simulink model "uGrid_1PH_hd_ATD2"  (R2018a)
settings: Solver=VariableStepAuto  StartTime=0.0  StopTime=.5  FixedStep=1e-6  MaxStep=1e-4  RelTol=1e-3
PreLoadFcn:
  | SimulinkInit
InitFcn:
  | SimulinkInit
StopFcn:
  | EndingScript
values from neighbouring files (symbols this model uses):
  ssAl = [-2.49999998232 0 0 0 376.789751319 0 -3.33333337039 0 0 376.789751319 0 0 ... (25 elements, 5x5)]    [modeloElectrico.mat]
  ssBl = [24.9999999997 0 0 0 0 0 33.333333333 0 0 0 0 0 ... (15 elements, 5x3)]    [modeloElectrico.mat]
  ssCl = [-0.229841748304 -0.00828937452901 0.991710625471 0 -0.229841748304 0.991710625471 -0.00828937452901 0 0.770158251696 -0.00828937452901 -0.00828937452901 0 ... (20 elements, 4x5)]    [modeloElectrico.mat]
  Tao1 = 0.5    [SimulinkInit.m]    (also in modeloDiesel_dotros.mat)
undefined symbols (not defined in the file or in its folder): G, GF, Ion, Lithium, ss1, ss2
libraries: powerlib x59, dsparch4 x12, truetime x12, powerlib_meascontrol x4, simulink x2, electricdrivelib x1
(part 1 of 2)
settings Model: Creator=erich  LastModifiedBy=cmparedes
settings CodeAppCC: StateflowObjectComments=on
settings SimscapeCC: SimscapeNormalizeSystem=off

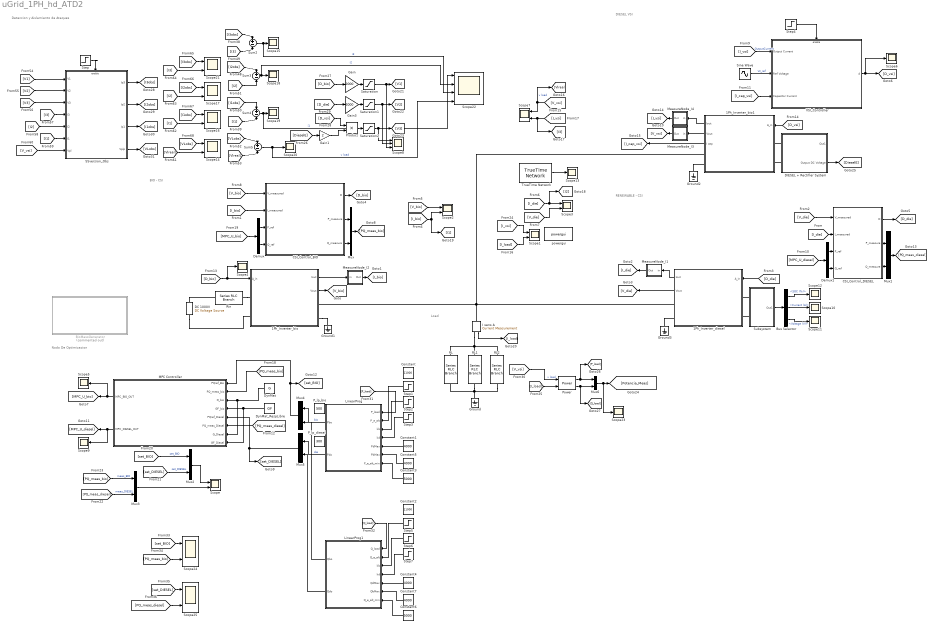
== system uGrid_1PH_hd_ATD2 ==
  note: Deteccion y Aislamiento de Ataques
  note: DIESEL VSI
  note: Load
  note: BIO - CSI
  note: RENEWABLE - CSI
  note: Nodo De Optimizacion
  1Ph_Inverter_bio : Subsystem  mask{st_time=0, f_sw=12000, samp_f=1e-6}
      mask prompts: st_time "Tiempo muerto (Start)"; f_sw "Switching frequency"; samp_f "samplig"
      mask Display:
      | port_label('input', 1, 'd', 'texmode', 'on')
      | 
      | port_label('lconn', 1, 'DC +')
      | port_label('lconn', 2, 'DC -')
      | 
      | 
      | port_label('rconn', 1, 'V_{out+}')
      | port_label('rconn', 2, 'B_{out-}')
      | 
      | 
      | port_label('output', 1, 'I_{out}', 'texmode', 'on')
      | port_label('output', 2, 'V_{out}', 'texmode', 'on')
      | 
      | plot([0.1 .9], [0.1 .9])
      | plot([0.2 .4], [.7 .7])
      | plot([0.2 .24], [.65 .65])
      | plot([0.28 .32], [.65 .65])
      | plot([0.36 .40], [.65 .65])
      | 
      | plot([.5:.01:.7], .25+sin(30*[.2:.01:.4])/10)
  1Ph_Inverter_bio1 : Subsystem  mask{st_time=0, f_sw=12000, samp_f=1e-6}
      mask prompts: st_time "Tiempo muerto (Start)"; f_sw "Switching frequency"; samp_f "samplig"
      mask Display:
      | port_label('input', 1, 'd', 'texmode', 'on')
      | 
      | port_label('lconn', 1, 'DC +')
      | port_label('lconn', 2, 'DC -')
      | 
      | 
      | port_label('rconn', 1, 'V_{out+}')
      | port_label('rconn', 2, 'B_{out-}')
      | 
      | 
      | port_label('output', 1, 'I_{out}', 'texmode', 'on')
      | port_label('output', 2, 'V_{out}', 'texmode', 'on')
      | port_label('output', 3, 'I_{cap}', 'texmode', 'on')
      | 
      | plot([0.1 .9], [0.1 .9])
      | plot([0.2 .4], [.7 .7])
      | plot([0.2 .24], [.65 .65])
      | plot([0.28 .32], [.65 .65])
      | plot([0.36 .40], [.65 .65])
      | 
      | plot([.5:.01:.7], .25+sin(30*[.2:.01:.4])/10)
  1Ph_Inverter_diesel : Subsystem  mask{st_time=0, f_sw=12000, samp_f=1e-6}
      mask prompts: st_time "Tiempo muerto (Start)"; f_sw "Switching frequency"; samp_f "Sampling frequency"
      mask Display:
      | port_label('input', 1, 'd', 'texmode', 'on')
      | 
      | port_label('lconn', 1, 'DC +')
      | port_label('lconn', 2, 'DC -')
      | 
      | 
      | port_label('rconn', 1, 'V_{out+}')
      | port_label('rconn', 2, 'B_{out-}')
      | 
      | 
      | port_label('output', 1, 'I_{out}', 'texmode', 'on')
      | port_label('output', 2, 'V_{out}', 'texmode', 'on')
      | 
      | plot([0.1 .9], [0.1 .9])
      | plot([0.2 .4], [.7 .7])
      | plot([0.2 .24], [.65 .65])
      | plot([0.28 .32], [.65 .65])
      | plot([0.36 .40], [.65 .65])
      | 
      | plot([.5:.01:.7], .25+sin(30*[.2:.01:.4])/10)
  BioMassGenerator : Subsystem  Commented=on
  Bus Selector : BusSelector  OutputSignals=SOC (%),Current (A),Voltage (V)
  CSI_Control_BIO : Subsystem
  CSI_Control_DIESEL : Subsystem
  Constant : Constant  Value=11000
  Constant{1,4..5,7} (4 alike) : Constant  Value=4000
  Constant2 : Constant  Value=11000
  Constant3 : Constant  Value=5000
  Constant6 : Constant  Value=5000
  DC 1000V : powerlib/Electrical Sources/DC Voltage Source  Amplitude=1000  Measurements=None
  DIESEL + Rectifier System : Subsystem
  Demux : Demux  Outputs=2
  Demux1 : Demux  Outputs=2
  DynMat : Constant  Value=G
  DynMat_RespLibre : Constant  Value=GF
  Gain : Gain  Gain=2000
  Gain1 : Gain  Gain=2
  Gain3 : Gain  Gain=2000
  Ground{,1..3} (4 alike) : powerlib/Elements/Ground  LConnTagsString=a
  I sens A : powerlib/Measurements/Current Measurement  PhasorSimulation=off  OutputType=Complex  PSBequivalent=0
  LinearProg : MATLAB Function  TreatAsAtomicUnit=on  SystemSampleTime=1e-3
  LinearProg1 : MATLAB Function  TreatAsAtomicUnit=on  SystemSampleTime=1e-3
  MPC Controller : Subsystem
  MeasureNode_I1 : Subsystem
  MeasureNode_I2 : Subsystem
  MeasureNode_I3 : Subsystem
  MeasureNode_I4 : Subsystem
  Mux{,1..6} (7 alike) : Mux  Inputs=2
  P_lp_bio : Constant  Value=500
  P_lp_diesel : Constant  Value=300
  Power : powerlib_meascontrol/Measurements/Power  Freq=60  Vinit=[1, 0]  Iinit=[1, 0]  Ts=0
      settings: SourceProductName=Simscape Power Systems
  Product : Product
  RL : powerlib/Elements/Series RLC Branch  LConnTagsString=__new0  RConnTagsString=__new0  BranchType=R  Resistance=10  Inductance=500e-3  SetiL0=off  InitialCurrent=0  Capacitance=100e-6  Setx0=off  InitialVoltage=0  Measurements=None
  RL1 : powerlib/Elements/Series RLC Branch  LConnTagsString=__new0  RConnTagsString=__new0  BranchType=RL  Resistance=10  Inductance=5.2  SetiL0=off  InitialCurrent=0  Capacitance=100e-6  Setx0=off  InitialVoltage=0  Measurements=None
  RL2 : powerlib/Elements/Series RLC Branch  LConnTagsString=__new0  RConnTagsString=__new0  BranchType=C  Resistance=30  Inductance=500e-3  SetiL0=off  InitialCurrent=0  Capacitance=2000e-6  Setx0=off  InitialVoltage=0  Measurements=None
  Rin : powerlib/Elements/Series RLC Branch  LConnTagsString=__new0  RConnTagsString=__new0  BranchType=R  Resistance=.001  Inductance=0  SetiL0=off  InitialCurrent=0  Capacitance=0  Setx0=off  InitialVoltage=0  Measurements=None
  SSversion_Obs : Subsystem
  Saturation : Saturate  UpperLimit=1000  LowerLimit=-1000
  Saturation1 : Saturate  UpperLimit=1000  LowerLimit=-1000
  Saturation2 : Saturate  UpperLimit=1000  LowerLimit=-1000
  Scope{,1..3,7,14,16..17,21,24..25} (11 alike) : Scope  NumInputPorts=2
  Scope{4..6,9..13,15,18..20,23} (13 alike) : Scope
  Scope22 : Scope  NumInputPorts=4
  Scope8 : Scope  NumInputPorts=3
  Sine Wave : Sin  Amplitude=170  Frequency=2*pi*60  SampleTime=0
  Step : Step  Time=0  SampleTime=0
  Step1 : Step  Time=0.3  Before=20000  After=5000  SampleTime=0
  Step2 : Step  Time=.6  Before=1.2  After=.4  SampleTime=0
  Step3 : Step  Before=.7  After=.7  SampleTime=0
  Step4 : Step  Time=10e-3  SampleTime=0
  Step5 : Step  Time=.3  Before=20000  After=5000  SampleTime=0
  Step6 : Step  Time=.6  Before=1.2  After=.4  SampleTime=0
  Step7 : Step  Before=.7  After=.7  SampleTime=0
  Subsystem : Subsystem
  Sum{2..5} (4 alike) : Sum  Inputs=+-
  TrueTime Network : truetime/TrueTime Network  nwtype=CSMA/CD (Ethernet)  nwnbr=1  nnodes=10  rate=8*1e9  minsize=512  lossprob=0  seed=0  bandwidths=[0.5 0.5]  slotsize=512  schedule=[1 1 2]  memsize=80000  buftype=Common buffer  overflow=Retransmit  dynSchedule=0  miniSlotSize=0  NIT=0  QSortMode=FIFO  sync=0  irtSchedule=0  nrtLength=0  nodeGraph=0  scheduleoutput=on
  VSI_Controller : Subsystem
  powergui : powerlib/powergui  Priority=1  SimulationMode=Continuous  SampleTime=50e-6  frequency=60  Iterations=50  frequencyindice=0  Pbase=100e6  ErrMax=1e-4  UnitsV=kV  UnitsW=MW  buscounter=0  FunctionMessages=off  echomessages=off  EnableUseOfTLC=off  CurrentSourceSwitches=off  DisableSnubberDevices=off  DisableRonSwitches=off  DisableVfSwitches=off  DisplayEquations=off  SolverType=Tustin/Backward Euler (TBE)  Interpol=off  ExternalGateDelay=off  methode=off  Ts=100  x0status=blocks  SPID=on  SwTol=0  HookPort=off  RestoreLinks=warning  ResistiveCurrentMeasurement=off  Frange=[0:2:500]  Ylog=off  Xlog=on  ShowGrid=off  save=off  variable=ZData  structure=0  ZoomFFT=off  StartTime=0.0  cycles=1  DisplayStyle=1  fundamental=60  FreqAxis=off  MaxFrequency=1000  frequencyindicesteady=1  RmsSteady=1  display=off
  wires:
  [D_bio] -> Scope4/1, 1Ph_Inverter_bio/1(A_in)
  [D_die] -> 1Ph_Inverter_diesel/1(A_in)
  [I_bio] -> [I1], Scope2/2
  [V_bio] -> Scope2/1
  [I_die] -> [I2], Scope3/1
  [V_die] -> Scope3/2
  1Ph_Inverter_bio/1(Iout) -> MeasureNode_I2/1(in)
  1Ph_Inverter_bio/2(Vout) -> [V_bio]
  1Ph_Inverter_diesel/1(Iout) -> MeasureNode_I1/1(in)
  1Ph_Inverter_diesel/2(Vout) -> [V_die]
  CSI_Control_BIO/1(D) -> [D_bio]
  [I_bio] -> CSI_Control_BIO/2(I_measured)
  [V_bio] -> CSI_Control_BIO/1(V_measured)
  CSI_Control_DIESEL/1(D) -> [D_die]
  [I_die] -> CSI_Control_DIESEL/2(I_measured)
  [V_die] -> CSI_Control_DIESEL/1(V_measured)
  [I_vsi] -> Scope1/1
  [I_load] -> Scope1/2
  Mux/1 -> [PQ_meas_bio]
  [MPC_U_bio] -> Demux/1
  [MPC_U_diesel] -> Demux1/1
  Mux1/1 -> [PQ_meas_diesel]
  [set_DIESEL] -> Mux2/2  "set_DIESEL"
  [set_BIO] -> Mux2/1  "set_BIO"
  Mux2/1 -> Scope/1
  Mux3/1 -> Scope/2
  [PQ_meas_diesel] -> Mux3/2  "meas_DIESEL"
  [PQ_meas_bio] -> Mux3/1  "meas_BIO"
  CSI_Control_BIO/2(P_measure) -> Mux/1
  CSI_Control_BIO/3(Q_measure) -> Mux/2
  CSI_Control_DIESEL/2(P_measure) -> Mux1/1
  CSI_Control_DIESEL/3(Q_measure) -> Mux1/2
  Demux1/1 -> CSI_Control_DIESEL/3(P_ref)
  Demux1/2 -> CSI_Control_DIESEL/4(Q_ref)
  Demux/1 -> CSI_Control_BIO/3(P_ref)
  Demux/2 -> CSI_Control_BIO/4(Q_ref)
  DynMat_RespLibre/1 -> MPC Controller/4(GF_bio), MPC Controller/8(GF_Diesel)
  DynMat/1 -> MPC Controller/3(G_bio), MPC Controller/7(G_Diesel)
  MPC Controller/2(MPC_DIESEL_OUT) -> [MPC_U_diesel], Scope9/1
  MPC Controller/1(MPC_BIO_OUT) -> Scope5/1, [MPC_U_bio]
  [PQ_meas_bio] -> MPC Controller/2(PQ_meas_bio)
  [PQ_meas_diesel] -> MPC Controller/6(PQ_meas_Diesel)
  Constant3/1 -> LinearProg/7(P_e_alt_min)
  Constant5/1 -> LinearProg/6(PbMax)
  Step2/1 -> LinearProg/3(kb)
  Step3/1 -> LinearProg/4(kd)
  Constant1/1 -> LinearProg/5(PdMax)
  Step1/1 -> LinearProg/2(P_e_alt)
  Mux5/1 -> [set_DIESEL], MPC Controller/5(PQref_Diesel)
  Mux4/1 -> MPC Controller/1(PQref_Bio), [set_BIO]
  VSI_Controller/1(d) -> Scope6/1, [D_vsi]
  [I_vsi] -> VSI_Controller/1(Output Current)  "OutputCurrent"
  Sine Wave/1 -> VSI_Controller/2(Ref Voltage)  "Vc_ref"
  [I_cap_vsi] -> VSI_Controller/3(Capacitor Current)
  1Ph_Inverter_bio1/3(I cap) -> [I_cap_vsi]
  [D_vsi] -> 1Ph_Inverter_bio1/1(A_in)
  1Ph_Inverter_bio1/2(Vout) -> MeasureNode_I3/1(in)
  [V_vsi] -> [Vlreal], Scope7/1  "v load"
  [I_vsi] -> [I3], Scope7/2
  [D_bio] -> Gain/1
  Gain/1 -> Saturation/1
  Saturation/1 -> [V1], Scope8/3
  Saturation1/1 -> Scope8/2, [V2]
  Saturation2/1 -> [V3], Scope8/1
  Product/1 -> Saturation2/1
  Sum2/1 -> Scope22/3, Scope15/1  "i3"
  [I3] -> Sum2/2
  Sum4/1 -> Scope22/1, Scope19/1  "i1"
  [VLobs] -> Sum5/1
  [I2obs] -> Sum3/1
  [I1] -> Sum4/2
  Sum3/1 -> Scope22/2, Scope18/1  "i2"
  [I1obs] -> Sum4/1
  [Vlreal] -> Sum5/2
  Sum5/1 -> Scope22/4, Scope20/1  "v load"
  [I2] -> Sum3/2
  [I3obs] -> Sum2/1
  [D_vsi] -> Product/1
  [V1] -> SSversion_Obs/1(V1)
  [V2] -> SSversion_Obs/2(V2)
  [V3] -> SSversion_Obs/3(V3)
  [I3] -> SSversion_Obs/4(I3)
  [I2] -> SSversion_Obs/5(I2)
  [I1] -> SSversion_Obs/6(I1)
  [V_vsi] -> SSversion_Obs/7(Vpl)
  [I3obs] -> Scope21/1
  [I2obs] -> Scope17/1
  [I2] -> Scope17/2
  [I1] -> Scope16/2
  [Vlreal] -> Scope14/2
  [VLobs] -> Scope14/1
  [I1obs] -> Scope16/1
  [I3] -> Scope21/2
  SSversion_Obs/1(Ip3) -> [I3obs]
  SSversion_Obs/2(Ip2) -> [I2obs]
  SSversion_Obs/3(Ip1) -> [I1obs]
  SSversion_Obs/4(Vplp) -> [VLobs]
  MeasureNode_I2/1(Out) -> [I_bio]
  MeasureNode_I1/1(Out) -> [I_die]
  MeasureNode_I4/1(Out) -> [I_vsi]
  1Ph_Inverter_bio1/1(Iout) -> MeasureNode_I4/1(in)
  I sens A/1 -> [I_load]
  MeasureNode_I3/1(Out) -> [V_vsi]
  [DieselE] -> Gain1/1
  Step/1 -> SSversion_Obs/Enable
  DIESEL + Rectifier System/2(Output DC Voltage) -> [DieselE]
  Bus Selector/2 -> Scope10/1  "<Current (A)>"
  Bus Selector/1 -> Scope12/1  "<SOC (%)>"
  Bus Selector/3 -> Scope11/1  "<Voltage (V)>"
  Subsystem/1(Out1) -> Bus Selector/1
  Step4/1 -> VSI_Controller/Enable
  Gain3/1 -> Saturation1/1
  [D_die] -> Gain3/1
  Gain1/1 -> Product/2
  TrueTime Network/1 -> Scope13/1
  Power/2 -> [Q_load], Mux6/2
  [I_load] -> Power/2
  Mux6/1 -> Scope23/1, [Potencia_Meas]
  [V_vsi] -> Power/1  "v load"
  Power/1 -> [P_load], Mux6/1
  Constant4/1 -> LinearProg1/5(QdMax)
  Step5/1 -> LinearProg1/2(Q_e_alt)
  Constant7/1 -> LinearProg1/6(QbMax)
  Step6/1 -> LinearProg1/3(kb)
  Step7/1 -> LinearProg1/4(kd)
  Constant6/1 -> LinearProg1/7(Q_e_alt_min)
  [P_load] -> LinearProg/1(P_load)
  [Q_load] -> LinearProg1/1(Q_load)
  LinearProg/1(Pbo) -> Mux4/1  "bio"
  LinearProg/2(Pdo) -> Mux5/1  "die"
  LinearProg1/1(Qbo) -> Mux4/2
  LinearProg1/2(Qdo) -> Mux5/2
  [set_BIO] -> Scope24/1
  [PQ_meas_bio] -> Scope24/2
  [set_DIESEL] -> Scope25/1
  [PQ_meas_diesel] -> Scope25/2
  connections:
  RL/LConn1 -- I sens A/RConn1 -- RL2/LConn1 -- RL1/LConn1
  Ground/LConn1 -- RL1/RConn1 -- RL2/RConn1 -- RL/RConn1
  1Ph_Inverter_bio/RConn2 -- Ground1/LConn1
  DC 1000V/LConn1 -- 1Ph_Inverter_bio/LConn2
  Rin/RConn1 -- 1Ph_Inverter_bio/LConn1
  1Ph_Inverter_diesel/RConn2 -- Ground3/LConn1
  1Ph_Inverter_diesel/RConn1 -- I sens A/LConn1 -- 1Ph_Inverter_bio/RConn1 -- 1Ph_Inverter_bio1/RConn1
  DC 1000V/RConn1 -- Rin/LConn1
  1Ph_Inverter_bio1/RConn2 -- Ground2/LConn1
  Subsystem/LConn1 -- 1Ph_Inverter_diesel/LConn1
  Subsystem/LConn2 -- 1Ph_Inverter_diesel/LConn2
  DIESEL + Rectifier System/LConn1 -- 1Ph_Inverter_bio1/LConn1
  DIESEL + Rectifier System/LConn2 -- 1Ph_Inverter_bio1/LConn2

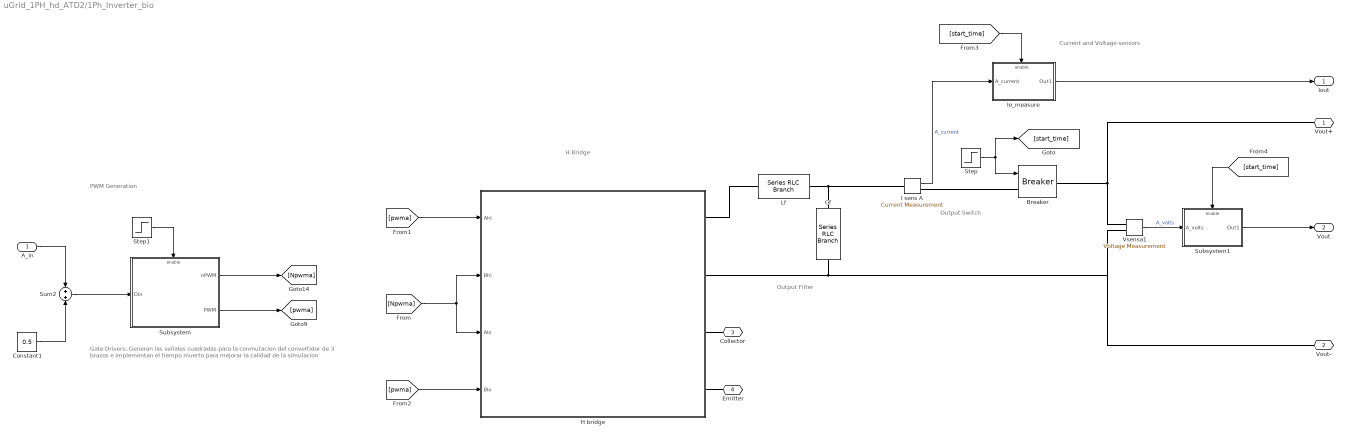
== system uGrid_1PH_hd_ATD2/1Ph_Inverter_bio ==
  note: PWM Generation
  note: H Bridge
  note: Output Filter
  note: Current and Voltage sensors
  note: Output Switch
  note: Gate Drivers: Generan las señales cuadradas para
      | la conmutacion del convertidor de 3 brazos e implementan el
      | tiempo muerto para mejorar la calidad de la simulacion
  A_in : Inport
  Breaker : powerlib/Elements/Breaker  InitialState=0  SwitchingTimes="[1/60  5/60]"  External=on  BreakerResistance=0.01  SnubberResistance=1e6  SnubberCapacitance=inf  Measurements=None  MoreParameters=on  NoBreakLoop=off
      settings: SourceProductName=Simscape Power Systems
  Cf : powerlib/Elements/Series RLC Branch  LConnTagsString=__new0  RConnTagsString=__new0  BranchType=C  Resistance=1  Inductance=1e-3  SetiL0=off  InitialCurrent=0  Capacitance=22e-6  Setx0=off  InitialVoltage=0  Measurements=None
  Constant1 : Constant  Value=0.5
  H bridge : Subsystem
      mask Display:
      | port_label('input', 1, '\fontsize{12} Ahi', 'texmode', 'on')
      | port_label('input', 2, '\fontsize{12} Alo', 'texmode', 'on')
      | port_label('input', 3, '\fontsize{12} Bhi', 'texmode', 'on')
      | port_label('input', 4, '\fontsize{12} Blo', 'texmode', 'on')
      | 
      | 
      | port_label('rconn', 1, '\fontsize{12} V_{out} +', 'texmode', 'on')
      | port_label('rconn', 2, '\fontsize{12} V_{out} -', 'texmode', 'on')
      | 
      | port_label('rconn', 3, '\fontsize{12} Collector', 'texmode', 'on')
      | port_label('rconn', 4, '\fontsize{12} Emitter', 'texmode', 'on')
      | 
      | lvx = [.1 .1];
      | lvy = [.1 .2];
      | lhx = [.1 .2];
      | lhy = [.1 .1];
      | 
      | 
      | % se dibujan los interruptores de la izquierda
      | plot(lvx+.07, lvy*.8+.028+.1)
      | plot(lvx+.1, lvy+.1)
      | plot(lhx*.5+.15, lhy+.1)
      | plot(lhx*.5+.15, lhy+.2)
      | plot(lhx*.5+.07, lhy+.15)
      | 
      | d=0.5;
      | 
      | plot(lvx+.07, lvy*.8+.028+.1+d)
      | plot(lvx+.1, lvy+.1+d)
      | plot(lhx*.5+.15, lhy+.1+d)
      | plot(lhx*.5+.15, lhy+.2+d)
      | plot(lhx*.5+.07, lhy+.15+d)
      | 
      | 
      | % se dibujan los interruptores del medio
      | h=.3;
      | 
      | %plot(lvx+.07+h, lvy*.8+.028+.1)
      | %plot(lvx+.1+h, lvy+.1)
      | %plot(lhx*.5+.15+h, lhy+.1)
      | %plot(lhx*.5+.15+h, lhy+.2)
      | %plot(lhx*.5+.07+h, lhy+.15)
      | 
      | %plot(lvx+.07+h, lvy*.8+.028+.1+d)
      | %plot(lvx+.1+h, lvy+.1+d)
      | %plot(lhx*.5+.15+h, lhy+.1+d)
      | %plot(lhx*.5+.15+h, lhy+.2+d)
      | %plot(lhx*.5+.07+h, lhy+.15+d)
      | 
      | % se dibujan los interruptores de la derecha
      | h=.6
      | 
      | plot(lvx+.07+h, lvy*.8+.028+.1)
      | plot(lvx+.1+h, lvy+.1)
      | plot(lhx*.5+.15+h, lhy+.1)
      | plot(lhx*.5+.15+h, lhy+.2)
      | plot(lhx*.5+.07+h, lhy+.15)
      | 
      | plot(lvx+.07+h, lvy*.8+.028+.1+d)
      | plot(lvx+.1+h, lvy+.1+d)
      | plot(lhx*.5+.15+h, lhy+.1+d)
      | plot(lhx*.5+.15+h, lhy+.2+d)
      | plot(lhx*.5+.07+h, lhy+.15+d)
      | 
      | 
      | % se conectan los interruptores.
      | plot(lvx+.15, lvy*4-.1)
      | %plot(lvx+.15+.3, lvy*4-.1)
      | plot(lvx+.15+.6, lvy*4-.1)
      | 
      | 
      | plot(lvx+.15, lvy+.7)
      | %plot(lvx+.15+.3, lvy+.7)
      | plot(lvx+.15+.6, lvy+.7)
      | 
      | plot(lvx+.15, lvy)
      | %plot(lvx+.15+.3, lvy)
      | plot(lvx+.15+.6, lvy)
      | 
      | plot(lhx*6-.35, lhy)
      | plot(lhx*6-.35, lhy+.8)
      | 
      | % raul esteban alzate 313 515 86 11
  I sens A : powerlib/Measurements/Current Measurement  PhasorSimulation=off  OutputType=Complex  PSBequivalent=0
  Io_measure : Subsystem
  Lf : powerlib/Elements/Series RLC Branch  LConnTagsString=__new0  RConnTagsString=__new0  BranchType=RL  Resistance=.1  Inductance=40e-3  SetiL0=off  InitialCurrent=0  Capacitance=1e-6  Setx0=off  InitialVoltage=0  Measurements=None
  Step : Step  Time=st_time  SampleTime=0
  Step1 : Step  Time=st_time  SampleTime=0
  Subsystem : Subsystem
  Subsystem1 : Subsystem
  Sum2 : Sum
  Vsensa1 : powerlib/Measurements/Voltage Measurement  PhasorSimulation=off  OutputType=Complex  PSBequivalent=0
  Vout+ : PMIOPort  Side=Right
  Vout- : PMIOPort  Port=2  Side=Right
  Collector : PMIOPort  Port=3  Side=Left
  Emitter : PMIOPort  Port=4  Side=Left
  Iout : Outport
  Vout : Outport  Port=2
  wires:
  Constant1/1 -> Sum2/2
  A_in/1 -> Sum2/1
  [pwma] -> H bridge/1(Ahi)
  [Npwma] -> H bridge/2(Bhi), H bridge/3(Alo)
  [pwma] -> H bridge/4(Blo)
  Step/1 -> [start_time], Breaker/1
  Sum2/1 -> Subsystem/1(Din)
  Subsystem/1(nPWM) -> [Npwma]
  Subsystem/2(PWM) -> [pwma]
  Step1/1 -> Subsystem/Enable
  I sens A/1 -> Io_measure/1(A_current)  "A_current"
  Io_measure/1(Out1) -> Iout/1
  [start_time] -> Io_measure/Enable
  Vsensa1/1 -> Subsystem1/1(A_volts)  "A_volts"
  Subsystem1/1(Out1) -> Vout/1
  [start_time] -> Subsystem1/Enable
  connections:
  H bridge/RConn3 -- Collector/RConn1
  H bridge/RConn4 -- Emitter/RConn1
  Lf/LConn1 -- H bridge/RConn1
  H bridge/RConn2 -- Vsensa1/LConn2 -- Vout-/RConn1 -- Cf/RConn1
  Breaker/LConn1 -- I sens A/RConn1
  Breaker/RConn1 -- Vout+/RConn1 -- Vsensa1/LConn1
  Cf/LConn1 -- I sens A/LConn1 -- Lf/RConn1

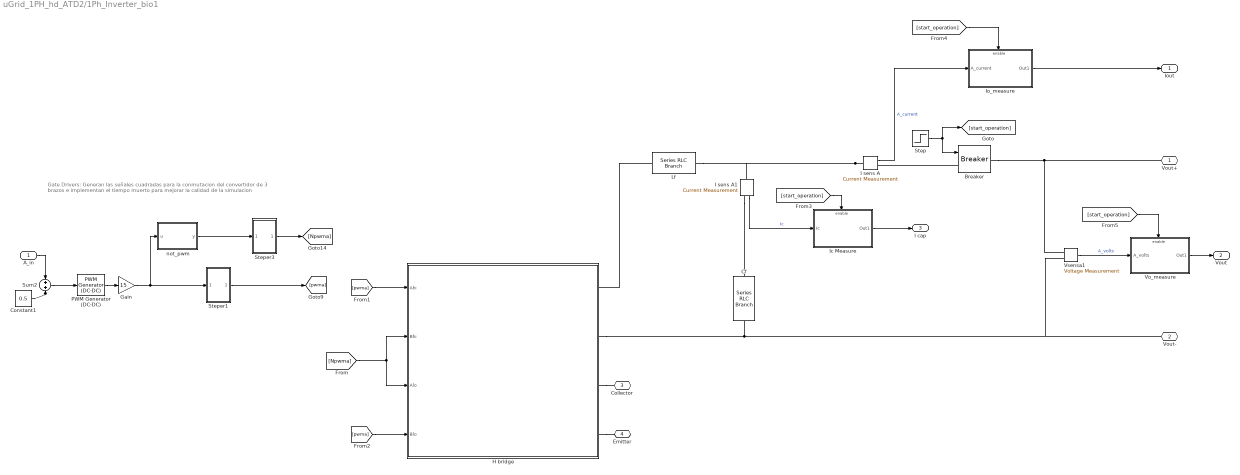
== system uGrid_1PH_hd_ATD2/1Ph_Inverter_bio1 ==
  note: Gate Drivers: Generan las señales cuadradas para
      | la conmutacion del convertidor de 3 brazos e implementan el
      | tiempo muerto para mejorar la calidad de la simulacion
  A_in : Inport
  Breaker : powerlib/Elements/Breaker  InitialState=0  SwitchingTimes="[1/60  5/60]"  External=on  BreakerResistance=0.01  SnubberResistance=1e6  SnubberCapacitance=inf  Measurements=None  MoreParameters=on  NoBreakLoop=off
      settings: SourceProductName=Simscape Power Systems
  Cf : powerlib/Elements/Series RLC Branch  LConnTagsString=__new0  RConnTagsString=__new0  BranchType=C  Resistance=1  Inductance=1e-3  SetiL0=off  InitialCurrent=0  Capacitance=610e-6  Setx0=off  InitialVoltage=0  Measurements=None
  Constant1 : Constant  Value=0.5
  Gain : Gain  Gain=15
  H bridge : Subsystem
      mask Display:
      | port_label('input', 1, '\fontsize{12} Ahi', 'texmode', 'on')
      | port_label('input', 2, '\fontsize{12} Alo', 'texmode', 'on')
      | port_label('input', 3, '\fontsize{12} Bhi', 'texmode', 'on')
      | port_label('input', 4, '\fontsize{12} Blo', 'texmode', 'on')
      | 
      | 
      | port_label('rconn', 1, '\fontsize{12} V_{out} +', 'texmode', 'on')
      | port_label('rconn', 2, '\fontsize{12} V_{out} -', 'texmode', 'on')
      | 
      | port_label('rconn', 3, '\fontsize{12} Collector', 'texmode', 'on')
      | port_label('rconn', 4, '\fontsize{12} Emitter', 'texmode', 'on')
      | 
      | lvx = [.1 .1];
      | lvy = [.1 .2];
      | lhx = [.1 .2];
      | lhy = [.1 .1];
      | 
      | 
      | % se dibujan los interruptores de la izquierda
      | plot(lvx+.07, lvy*.8+.028+.1)
      | plot(lvx+.1, lvy+.1)
      | plot(lhx*.5+.15, lhy+.1)
      | plot(lhx*.5+.15, lhy+.2)
      | plot(lhx*.5+.07, lhy+.15)
      | 
      | d=0.5;
      | 
      | plot(lvx+.07, lvy*.8+.028+.1+d)
      | plot(lvx+.1, lvy+.1+d)
      | plot(lhx*.5+.15, lhy+.1+d)
      | plot(lhx*.5+.15, lhy+.2+d)
      | plot(lhx*.5+.07, lhy+.15+d)
      | 
      | 
      | % se dibujan los interruptores del medio
      | h=.3;
      | 
      | %plot(lvx+.07+h, lvy*.8+.028+.1)
      | %plot(lvx+.1+h, lvy+.1)
      | %plot(lhx*.5+.15+h, lhy+.1)
      | %plot(lhx*.5+.15+h, lhy+.2)
      | %plot(lhx*.5+.07+h, lhy+.15)
      | 
      | %plot(lvx+.07+h, lvy*.8+.028+.1+d)
      | %plot(lvx+.1+h, lvy+.1+d)
      | %plot(lhx*.5+.15+h, lhy+.1+d)
      | %plot(lhx*.5+.15+h, lhy+.2+d)
      | %plot(lhx*.5+.07+h, lhy+.15+d)
      | 
      | % se dibujan los interruptores de la derecha
      | h=.6
      | 
      | plot(lvx+.07+h, lvy*.8+.028+.1)
      | plot(lvx+.1+h, lvy+.1)
      | plot(lhx*.5+.15+h, lhy+.1)
      | plot(lhx*.5+.15+h, lhy+.2)
      | plot(lhx*.5+.07+h, lhy+.15)
      | 
      | plot(lvx+.07+h, lvy*.8+.028+.1+d)
      | plot(lvx+.1+h, lvy+.1+d)
      | plot(lhx*.5+.15+h, lhy+.1+d)
      | plot(lhx*.5+.15+h, lhy+.2+d)
      | plot(lhx*.5+.07+h, lhy+.15+d)
      | 
      | 
      | % se conectan los interruptores.
      | plot(lvx+.15, lvy*4-.1)
      | %plot(lvx+.15+.3, lvy*4-.1)
      | plot(lvx+.15+.6, lvy*4-.1)
      | 
      | 
      | plot(lvx+.15, lvy+.7)
      | %plot(lvx+.15+.3, lvy+.7)
      | plot(lvx+.15+.6, lvy+.7)
      | 
      | plot(lvx+.15, lvy)
      | %plot(lvx+.15+.3, lvy)
      | plot(lvx+.15+.6, lvy)
      | 
      | plot(lhx*6-.35, lhy)
      | plot(lhx*6-.35, lhy+.8)
      | 
      | % raul esteban alzate 313 515 86 11
  I sens A : powerlib/Measurements/Current Measurement  PhasorSimulation=off  OutputType=Complex  PSBequivalent=0
  I sens A1 : powerlib/Measurements/Current Measurement  PhasorSimulation=off  OutputType=Complex  PSBequivalent=0
  Ic Measure : Subsystem
  Io_measure : Subsystem
  Lf : powerlib/Elements/Series RLC Branch  LConnTagsString=__new0  RConnTagsString=__new0  BranchType=RL  Resistance=1e-3  Inductance=5e-3  SetiL0=off  InitialCurrent=0  Capacitance=1e-6  Setx0=off  InitialVoltage=0  Measurements=None
  PWM Generator (DC-DC) : powerlib_meascontrol/Pulse & Signal Generators/PWM Generator (DC-DC)  Fsw=f_sw  Ts=samp_f
  Step : Step  Time=st_time  SampleTime=0
  Steper1 : Subsystem
  Steper3 : Subsystem
  Sum2 : Sum
  Vo_measure : Subsystem
  Vsensa1 : powerlib/Measurements/Voltage Measurement  PhasorSimulation=off  OutputType=Complex  PSBequivalent=0
  not_pwm : MATLAB Function  TreatAsAtomicUnit=on
  Vout+ : PMIOPort  Side=Right
  Vout- : PMIOPort  Port=2  Side=Right
  Collector : PMIOPort  Port=3  Side=Left
  Emitter : PMIOPort  Port=4  Side=Left
  Iout : Outport
  Vout : Outport  Port=2
  I cap : Outport  Port=3
  wires:
  not_pwm/1(y) -> Steper3/1(In1)
  Sum2/1 -> PWM Generator (DC-DC)/1
  PWM Generator (DC-DC)/1 -> Gain/1
  Constant1/1 -> Sum2/2
  A_in/1 -> Sum2/1
  Steper1/1(Out1) -> [pwma]
  Steper3/1(Out1) -> [Npwma]
  Gain/1 -> Steper1/1(In1), not_pwm/1(u)
  [pwma] -> H bridge/1(Ahi)
  [Npwma] -> H bridge/2(Bhi), H bridge/3(Alo)
  [pwma] -> H bridge/4(Blo)
  Step/1 -> [start_operation], Breaker/1
  I sens A1/1 -> Ic Measure/1(Ic)  "Ic"
  Ic Measure/1(Out1) -> I cap/1
  [start_operation] -> Ic Measure/Enable
  Vsensa1/1 -> Vo_measure/1(A_volts)  "A_volts"
  Vo_measure/1(Out1) -> Vout/1
  I sens A/1 -> Io_measure/1(A_current)  "A_current"
  Io_measure/1(Out1) -> Iout/1
  [start_operation] -> Io_measure/Enable
  [start_operation] -> Vo_measure/Enable
  connections:
  H bridge/RConn3 -- Collector/RConn1
  H bridge/RConn4 -- Emitter/RConn1
  Lf/LConn1 -- H bridge/RConn1
  H bridge/RConn2 -- Vout-/RConn1 -- Vsensa1/LConn2 -- Cf/RConn1
  Breaker/LConn1 -- I sens A/RConn1
  Breaker/RConn1 -- Vsensa1/LConn1 -- Vout+/RConn1
  I sens A/LConn1 -- Lf/RConn1 -- I sens A1/LConn1
  I sens A1/RConn1 -- Cf/LConn1

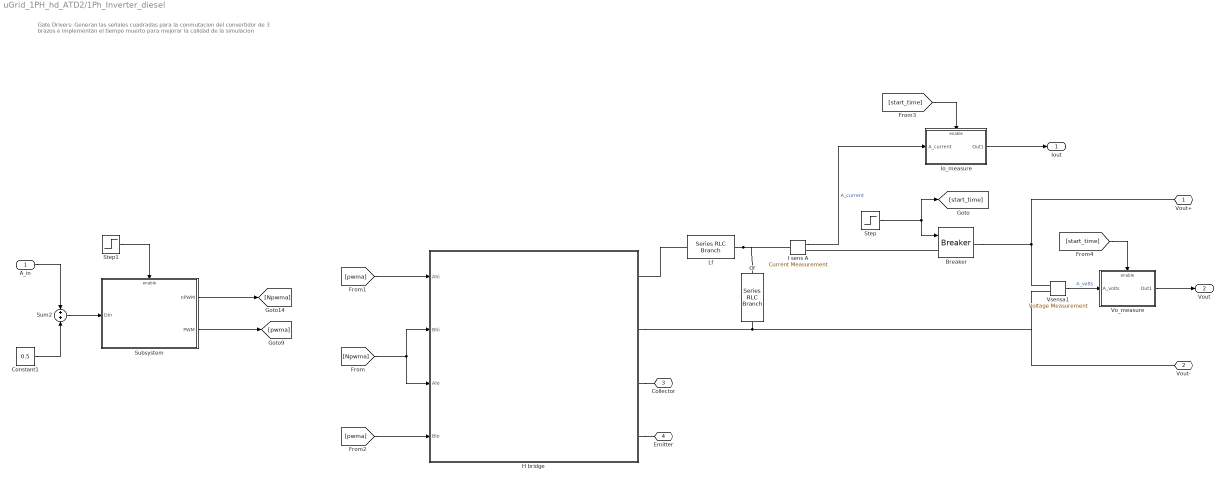
== system uGrid_1PH_hd_ATD2/1Ph_Inverter_diesel ==
  note: Gate Drivers: Generan las señales cuadradas para
      | la conmutacion del convertidor de 3 brazos e implementan el
      | tiempo muerto para mejorar la calidad de la simulacion
  A_in : Inport
  Breaker : powerlib/Elements/Breaker  InitialState=0  SwitchingTimes="[1/60  5/60]"  External=on  BreakerResistance=0.01  SnubberResistance=1e6  SnubberCapacitance=inf  Measurements=None  MoreParameters=on  NoBreakLoop=off
      settings: SourceProductName=Simscape Power Systems
  Cf : powerlib/Elements/Series RLC Branch  LConnTagsString=__new0  RConnTagsString=__new0  BranchType=C  Resistance=1  Inductance=1e-3  SetiL0=off  InitialCurrent=0  Capacitance=22e-6  Setx0=off  InitialVoltage=0  Measurements=None
  Constant1 : Constant  Value=0.5
  H bridge : Subsystem
      mask Display:
      | port_label('input', 1, '\fontsize{12} Ahi', 'texmode', 'on')
      | port_label('input', 2, '\fontsize{12} Alo', 'texmode', 'on')
      | port_label('input', 3, '\fontsize{12} Bhi', 'texmode', 'on')
      | port_label('input', 4, '\fontsize{12} Blo', 'texmode', 'on')
      | 
      | 
      | port_label('rconn', 1, '\fontsize{12} V_{out} +', 'texmode', 'on')
      | port_label('rconn', 2, '\fontsize{12} V_{out} -', 'texmode', 'on')
      | 
      | port_label('rconn', 3, '\fontsize{12} Collector', 'texmode', 'on')
      | port_label('rconn', 4, '\fontsize{12} Emitter', 'texmode', 'on')
      | 
      | lvx = [.1 .1];
      | lvy = [.1 .2];
      | lhx = [.1 .2];
      | lhy = [.1 .1];
      | 
      | 
      | % se dibujan los interruptores de la izquierda
      | plot(lvx+.07, lvy*.8+.028+.1)
      | plot(lvx+.1, lvy+.1)
      | plot(lhx*.5+.15, lhy+.1)
      | plot(lhx*.5+.15, lhy+.2)
      | plot(lhx*.5+.07, lhy+.15)
      | 
      | d=0.5;
      | 
      | plot(lvx+.07, lvy*.8+.028+.1+d)
      | plot(lvx+.1, lvy+.1+d)
      | plot(lhx*.5+.15, lhy+.1+d)
      | plot(lhx*.5+.15, lhy+.2+d)
      | plot(lhx*.5+.07, lhy+.15+d)
      | 
      | 
      | % se dibujan los interruptores del medio
      | h=.3;
      | 
      | %plot(lvx+.07+h, lvy*.8+.028+.1)
      | %plot(lvx+.1+h, lvy+.1)
      | %plot(lhx*.5+.15+h, lhy+.1)
      | %plot(lhx*.5+.15+h, lhy+.2)
      | %plot(lhx*.5+.07+h, lhy+.15)
      | 
      | %plot(lvx+.07+h, lvy*.8+.028+.1+d)
      | %plot(lvx+.1+h, lvy+.1+d)
      | %plot(lhx*.5+.15+h, lhy+.1+d)
      | %plot(lhx*.5+.15+h, lhy+.2+d)
      | %plot(lhx*.5+.07+h, lhy+.15+d)
      | 
      | % se dibujan los interruptores de la derecha
      | h=.6
      | 
      | plot(lvx+.07+h, lvy*.8+.028+.1)
      | plot(lvx+.1+h, lvy+.1)
      | plot(lhx*.5+.15+h, lhy+.1)
      | plot(lhx*.5+.15+h, lhy+.2)
      | plot(lhx*.5+.07+h, lhy+.15)
      | 
      | plot(lvx+.07+h, lvy*.8+.028+.1+d)
      | plot(lvx+.1+h, lvy+.1+d)
      | plot(lhx*.5+.15+h, lhy+.1+d)
      | plot(lhx*.5+.15+h, lhy+.2+d)
      | plot(lhx*.5+.07+h, lhy+.15+d)
      | 
      | 
      | % se conectan los interruptores.
      | plot(lvx+.15, lvy*4-.1)
      | %plot(lvx+.15+.3, lvy*4-.1)
      | plot(lvx+.15+.6, lvy*4-.1)
      | 
      | 
      | plot(lvx+.15, lvy+.7)
      | %plot(lvx+.15+.3, lvy+.7)
      | plot(lvx+.15+.6, lvy+.7)
      | 
      | plot(lvx+.15, lvy)
      | %plot(lvx+.15+.3, lvy)
      | plot(lvx+.15+.6, lvy)
      | 
      | plot(lhx*6-.35, lhy)
      | plot(lhx*6-.35, lhy+.8)
      | 
      | % raul esteban alzate 313 515 86 11
  I sens A : powerlib/Measurements/Current Measurement  PhasorSimulation=off  OutputType=Complex  PSBequivalent=0
  Io_measure : Subsystem
  Lf : powerlib/Elements/Series RLC Branch  LConnTagsString=__new0  RConnTagsString=__new0  BranchType=RL  Resistance=.1  Inductance=30e-3  SetiL0=off  InitialCurrent=0  Capacitance=1e-6  Setx0=off  InitialVoltage=0  Measurements=None
  Step : Step  Time=st_time  SampleTime=0
  Step1 : Step  Time=st_time  SampleTime=0
  Subsystem : Subsystem
  Sum2 : Sum
  Vo_measure : Subsystem
  Vsensa1 : powerlib/Measurements/Voltage Measurement  PhasorSimulation=off  OutputType=Complex  PSBequivalent=0
  Vout+ : PMIOPort  Side=Right
  Vout- : PMIOPort  Port=2  Side=Right
  Collector : PMIOPort  Port=3  Side=Left
  Emitter : PMIOPort  Port=4  Side=Left
  Iout : Outport
  Vout : Outport  Port=2
  wires:
  [pwma] -> H bridge/4(Blo)
  [Npwma] -> H bridge/3(Alo), H bridge/2(Bhi)
  [pwma] -> H bridge/1(Ahi)
  A_in/1 -> Sum2/1
  Constant1/1 -> Sum2/2
  Step/1 -> [start_time], Breaker/1
  Sum2/1 -> Subsystem/1(Din)
  Subsystem/1(nPWM) -> [Npwma]
  Subsystem/2(PWM) -> [pwma]
  Step1/1 -> Subsystem/Enable
  Vsensa1/1 -> Vo_measure/1(A_volts)  "A_volts"
  Vo_measure/1(Out1) -> Vout/1
  I sens A/1 -> Io_measure/1(A_current)  "A_current"
  Io_measure/1(Out1) -> Iout/1
  [start_time] -> Io_measure/Enable
  [start_time] -> Vo_measure/Enable
  connections:
  Cf/RConn1 -- Vsensa1/LConn2 -- Vout-/RConn1 -- H bridge/RConn2
  Lf/LConn1 -- H bridge/RConn1
  H bridge/RConn4 -- Emitter/RConn1
  H bridge/RConn3 -- Collector/RConn1
  Breaker/LConn1 -- I sens A/RConn1
  Breaker/RConn1 -- Vsensa1/LConn1 -- Vout+/RConn1
  Lf/RConn1 -- I sens A/LConn1 -- Cf/LConn1

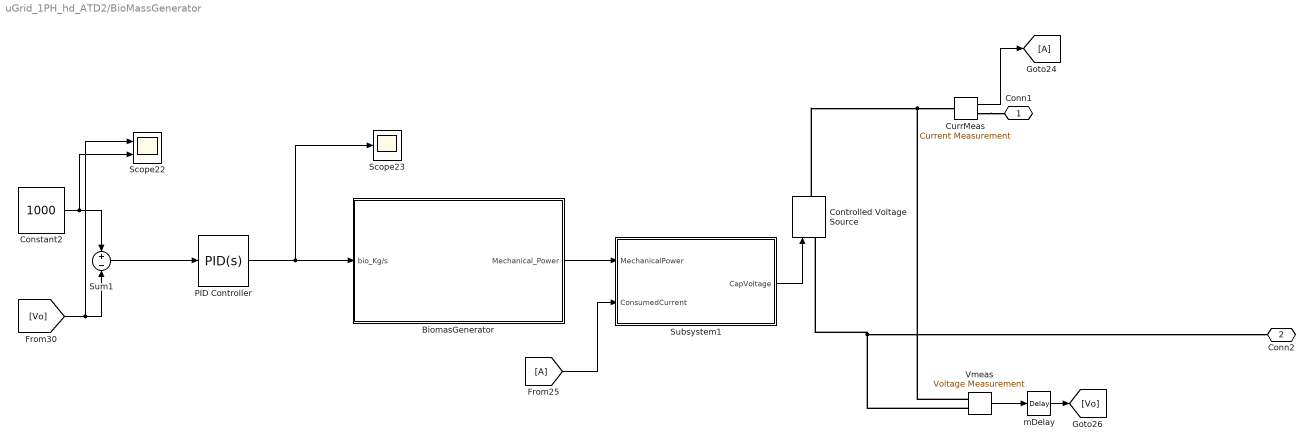
== system uGrid_1PH_hd_ATD2/BioMassGenerator ==
  BiomasGenerator : Subsystem
  Constant2 : Constant  Value=1000
  Controlled Voltage Source : powerlib/Electrical Sources/Controlled Voltage Source  Initialize=on  Source_Type=AC  Amplitude=0  Phase=0  Frequency=0  Measurements=None
  CurrMeas : powerlib/Measurements/Current Measurement  PhasorSimulation=off  OutputType=Complex  PSBequivalent=0
  PID Controller : simulink/Continuous/PID Controller  Controller=PID  TimeDomain=Continuous-time  SampleTime=-1  IntegratorMethod=Forward Euler  FilterMethod=Forward Euler  Form=Parallel  UseFilter=on  ControllerParametersSource=internal  P=.00012  I=.00004  D=0  N=100  InitialConditionSource=internal  InitialConditionForIntegrator=0  InitialConditionForFilter=0  ExternalReset=none  LimitOutput=off  UpperSaturationLimit=inf  LowerSaturationLimit=-inf  LinearizeAsGain=on  AntiWindupMode=none  Kb=1  TrackingMode=off  Kt=1  PParamMin=[]  PParamMax=[]  IParamMin=[]  IParamMax=[]  DParamMin=[]  DParamMax=[]  NParamMin=[]  NParamMax=[]  KbParamMin=[]  KbParamMax=[]  KtParamMin=[]  KtParamMax=[]  POutMin=[]  POutMax=[]  IOutMin=[]  IOutMax=[]  DOutMin=[]  DOutMax=[]  NOutMin=[]  NOutMax=[]  KbOutMin=[]  KbOutMax=[]  KtOutMin=[]  KtOutMax=[]  IntegratorOutMin=[]  IntegratorOutMax=[]  FilterOutMin=[]  FilterOutMax=[]  SumOutMin=[]  SumOutMax=[]  SumI1OutMin=[]  SumI1OutMax=[]  SumI2OutMin=[]  SumI2OutMax=[]  SumI3OutMin=[]  SumI3OutMax=[]  SumDOutMin=[]  SumDOutMax=[]  SaturationOutMin=[]  SaturationOutMax=[]  IntegratorContinuousStateAttributes=''  IntegratorStateMustResolveToSignalObject=off  IntegratorRTWStateStorageClass=Auto  FilterContinuousStateAttributes=''  FilterStateMustResolveToSignalObject=off  FilterRTWStateStorageClass=Auto  DifferentiatorICPrevScaledInput=0  DifferentiatorOutMin=[]  DifferentiatorOutMax=[]  FilterDiffOutCoefMin=[]  FilterDiffOutCoefMax=[]  SumDenOutMin=[]  SumDenOutMax=[]  SumNumOutMin=[]  SumNumOutMax=[]  ReciprocalOutMin=[]  ReciprocalOutMax=[]  DivideOutMin=[]  DivideOutMax=[]  TunerSelectOption=Transfer Function Based (PID Tuner App)
  Scope22 : Scope  NumInputPorts=2
  Scope23 : Scope
  Subsystem1 : Subsystem
  Sum1 : Sum  Inputs=+-
  Vmeas : powerlib/Measurements/Voltage Measurement  PhasorSimulation=off  OutputType=Complex  PSBequivalent=0
  mDelay : TransportDelay  DelayTime=1e-3
  Conn1 : PMIOPort  Side=Right
  Conn2 : PMIOPort  Port=2  Side=Right
  wires:
  CurrMeas/1 -> [A]
  PID Controller/1 -> BiomasGenerator/1(bio_Kg/s), Scope23/1
  [Vo] -> Sum1/2, Scope22/1
  mDelay/1 -> [Vo]
  [A] -> Subsystem1/2(ConsumedCurrent)
  BiomasGenerator/1(Mechanical_Power) -> Subsystem1/1(MechanicalPower)
  Subsystem1/1(CapVoltage) -> Controlled Voltage Source/1
  Constant2/1 -> Scope22/2, Sum1/1
  Vmeas/1 -> mDelay/1
  Sum1/1 -> PID Controller/1
  connections:
  Vmeas/LConn2 -- Controlled Voltage Source/LConn1 -- Conn2/RConn1
  Vmeas/LConn1 -- Controlled Voltage Source/RConn1 -- CurrMeas/LConn1
  CurrMeas/RConn1 -- Conn1/RConn1

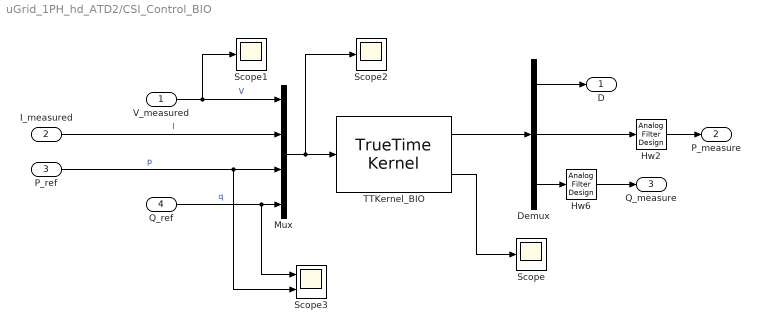
== system uGrid_1PH_hd_ATD2/CSI_Control_BIO ==
  V_measured : Inport
  I_measured : Inport  Port=2
  P_ref : Inport  Port=3
  Q_ref : Inport  Port=4
  Demux : Demux  Outputs=3
  Hw2 : dsparch4/Analog Filter Design  method=Bessel  filttype=Lowpass  N=4  Wlo=30*2*pi  Whi=80  Rp=2  Rs=80
  Hw6 : dsparch4/Analog Filter Design  method=Bessel  filttype=Lowpass  N=4  Wlo=30*2*pi  Whi=80  Rp=2  Rs=80
  Mux : Mux
  Scope : Scope
  Scope1 : Scope
  Scope2 : Scope
  Scope3 : Scope  NumInputPorts=2
  TTKernel_BIO : truetime/TrueTime Kernel  sfun=BIO_init  args=1  ninputsoutputs=[4 3]  ntriggers=0  trigtype=falling  nwnodenbr=[]  clockoffsetdrift=[0 0]  schedoutput=on  battery=off  poweroutput=off
  D : Outport
  P_measure : Outport  Port=2
  Q_measure : Outport  Port=3
  wires:
  TTKernel_BIO/1 -> Demux/1
  Demux/3 -> Hw6/1
  Demux/2 -> Hw2/1
  Demux/1 -> D/1
  TTKernel_BIO/2 -> Scope/1
  Mux/1 -> Scope2/1, TTKernel_BIO/1
  V_measured/1 -> Scope1/1, Mux/1  "V"
  I_measured/1 -> Mux/2  "I"
  P_ref/1 -> Scope3/2, Mux/3  "p"
  Q_ref/1 -> Scope3/1, Mux/4  "q"
  Hw6/1 -> Q_measure/1
  Hw2/1 -> P_measure/1

== system uGrid_1PH_hd_ATD2/CSI_Control_DIESEL ==
  V_measured : Inport
  I_measured : Inport  Port=2
  P_ref : Inport  Port=3
  Q_ref : Inport  Port=4
  Demux : Demux  Outputs=3
  Hw1 : dsparch4/Analog Filter Design  method=Bessel  filttype=Lowpass  N=4  Wlo=30*2*pi  Whi=80  Rp=2  Rs=80
  Hw3 : dsparch4/Analog Filter Design  method=Bessel  filttype=Lowpass  N=4  Wlo=30*2*pi  Whi=80  Rp=2  Rs=80
  Mux : Mux
  TTKernel_DIESEL : truetime/TrueTime Kernel  sfun=DIESEL_init  args=[]  ninputsoutputs=[4 3]  ntriggers=0  trigtype=falling  nwnodenbr=[]  clockoffsetdrift=[0 0]  schedoutput=on  battery=off  poweroutput=off
  D : Outport
  P_measure : Outport  Port=2
  Q_measure : Outport  Port=3
  wires:
  Mux/1 -> TTKernel_DIESEL/1
  Demux/3 -> Hw3/1
  Demux/2 -> Hw1/1
  TTKernel_DIESEL/1 -> Demux/1
  Demux/1 -> D/1
  Hw1/1 -> P_measure/1
  Hw3/1 -> Q_measure/1
  P_ref/1 -> Mux/3
  Q_ref/1 -> Mux/4
  I_measured/1 -> Mux/2
  V_measured/1 -> Mux/1

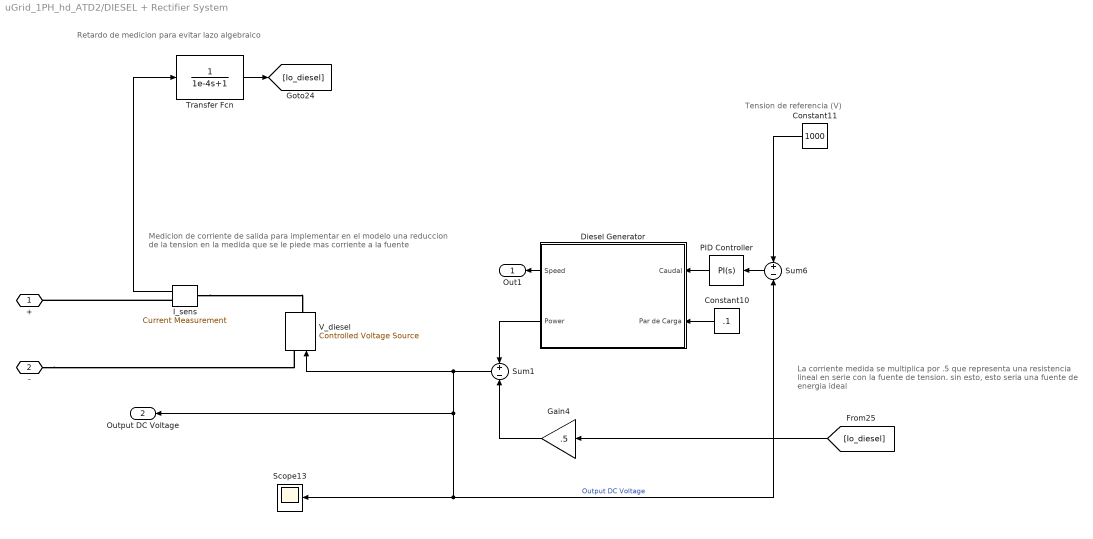
== system uGrid_1PH_hd_ATD2/DIESEL + Rectifier System ==
  note: Tension de referencia (V)
  note: La corriente medida se multiplica por .5 que
      | representa una resistencia lineal en serie con
      | la fuente de tension. sin esto, esto seria una
      | fuente de energia ideal
  note: Medicion de corriente de salida para implementar
      | en el modelo una reduccion de la tension en la
      | medida que se le piede mas corriente a la fuente
  note: Retardo de medicion para evitar lazo algebraico
  Constant10 : Constant  Value=.1
  Constant11 : Constant  Value=1000
  Diesel Generator : Subsystem
  Gain4 : Gain  Gain=.5
  I_sens : powerlib/Measurements/Current Measurement  PhasorSimulation=off  OutputType=Complex  PSBequivalent=0
  PID Controller : simulink/Continuous/PID Controller  Controller=PI  TimeDomain=Continuous-time  SampleTime=-1  IntegratorMethod=Forward Euler  FilterMethod=Forward Euler  Form=Parallel  UseFilter=on  ControllerParametersSource=internal  P=0.00325909628031494  I=0.000326732379168699  D=0.00124823483730586  N=0.606508283225141  InitialConditionSource=internal  InitialConditionForIntegrator=0.248  InitialConditionForFilter=0.24  ExternalReset=none  LimitOutput=off  UpperSaturationLimit=inf  LowerSaturationLimit=-inf  LinearizeAsGain=on  AntiWindupMode=none  Kb=1  TrackingMode=off  Kt=1  PParamMin=[]  PParamMax=[]  IParamMin=[]  IParamMax=[]  DParamMin=[]  DParamMax=[]  NParamMin=[]  NParamMax=[]  KbParamMin=[]  KbParamMax=[]  KtParamMin=[]  KtParamMax=[]  POutMin=[]  POutMax=[]  IOutMin=[]  IOutMax=[]  DOutMin=[]  DOutMax=[]  NOutMin=[]  NOutMax=[]  KbOutMin=[]  KbOutMax=[]  KtOutMin=[]  KtOutMax=[]  IntegratorOutMin=[]  IntegratorOutMax=[]  FilterOutMin=[]  FilterOutMax=[]  SumOutMin=[]  SumOutMax=[]  SumI1OutMin=[]  SumI1OutMax=[]  SumI2OutMin=[]  SumI2OutMax=[]  SumI3OutMin=[]  SumI3OutMax=[]  SumDOutMin=[]  SumDOutMax=[]  SaturationOutMin=[]  SaturationOutMax=[]  IntegratorContinuousStateAttributes=''  IntegratorStateMustResolveToSignalObject=off  IntegratorRTWStateStorageClass=Auto  FilterContinuousStateAttributes=''  FilterStateMustResolveToSignalObject=off  FilterRTWStateStorageClass=Auto  DifferentiatorICPrevScaledInput=0  DifferentiatorOutMin=[]  DifferentiatorOutMax=[]  InitialConditionSetting=State (most efficient)  FilterDiffOutCoefMin=[]  FilterDiffOutCoefMax=[]  SumDenOutMin=[]  SumDenOutMax=[]  SumNumOutMin=[]  SumNumOutMax=[]  ReciprocalOutMin=[]  ReciprocalOutMax=[]  DivideOutMin=[]  DivideOutMax=[]  TunerSelectOption=Transfer Function Based (PID Tuner App)
  Scope13 : Scope
  Sum1 : Sum  Inputs=+-
  Sum6 : Sum  Inputs=+-
  Transfer Fcn : TransferFcn  Denominator=[1e-4 1]
  V_diesel : powerlib/Electrical Sources/Controlled Voltage Source  Initialize=on  Source_Type=AC  Amplitude=0  Phase=0  Frequency=0  Measurements=None
  + : PMIOPort  Side=Left
  - : PMIOPort  Port=2  Side=Left
  Out1 : Outport
  Output DC Voltage : Outport  Port=2
  wires:
  Sum1/1 -> Output DC Voltage/1, Sum6/2, Scope13/1, V_diesel/1  "Output DC Voltage"
  Transfer Fcn/1 -> [Io_diesel]
  I_sens/1 -> Transfer Fcn/1
  Diesel Generator/2(Power) -> Sum1/1
  Sum6/1 -> PID Controller/1
  Diesel Generator/1(Speed) -> Out1/1
  Gain4/1 -> Sum1/2
  Constant10/1 -> Diesel Generator/2(Par de Carga)
  Constant11/1 -> Sum6/1
  [Io_diesel] -> Gain4/1
  PID Controller/1 -> Diesel Generator/1(Caudal)
  connections:
  -/RConn1 -- V_diesel/LConn1
  I_sens/LConn1 -- V_diesel/RConn1
  I_sens/RConn1 -- +/RConn1

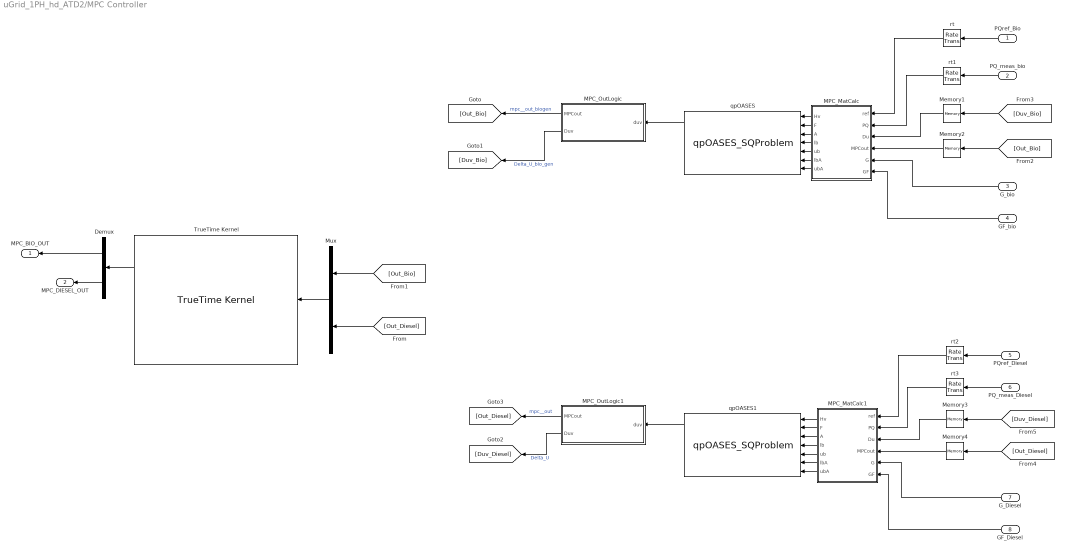
== system uGrid_1PH_hd_ATD2/MPC Controller ==
  PQref_Bio : Inport
  PQ_meas_bio : Inport  Port=2
  G_bio : Inport  Port=3
  GF_bio : Inport  Port=4
  PQref_Diesel : Inport  Port=5
  PQ_meas_Diesel : Inport  Port=6
  G_Diesel : Inport  Port=7
  GF_Diesel : Inport  Port=8
  Demux : Demux  Outputs=2
  MPC_MatCalc : MATLAB Function  TreatAsAtomicUnit=on  SystemSampleTime=1e-3
      settings: MinAlgLoopOccurrences=on
  MPC_MatCalc1 : MATLAB Function  TreatAsAtomicUnit=on  SystemSampleTime=1e-3
      settings: MinAlgLoopOccurrences=on
  MPC_OutLogic : MATLAB Function  TreatAsAtomicUnit=on
      settings: MinAlgLoopOccurrences=on
  MPC_OutLogic1 : MATLAB Function  TreatAsAtomicUnit=on
      settings: MinAlgLoopOccurrences=on
  Memory{1..4} (4 alike) : Memory
  Mux : Mux  Inputs=2
  TrueTime Kernel : truetime/TrueTime Kernel  sfun=MPC_PQ_init  args=[]  ninputsoutputs=[4 4]  ntriggers=0  trigtype=falling  nwnodenbr=[]  clockoffsetdrift=[0 0]  schedoutput=on  battery=off  poweroutput=off
  qpOASES : S-Function  FunctionName=qpOASES_SQProblem  SFunctionDeploymentMode=off  EnableBusSupport=off
  qpOASES1 : S-Function  FunctionName=qpOASES_SQProblem  SFunctionDeploymentMode=off  EnableBusSupport=off
  rt{,1..3} (4 alike) : RateTransition  InitialCondition=[0 0]  OutPortSampleTime=1e-3
  MPC_BIO_OUT : Outport
  MPC_DIESEL_OUT : Outport  Port=2
  wires:
  MPC_MatCalc/7(ubA) -> qpOASES/7
  G_bio/1 -> MPC_MatCalc/5(G)
  MPC_MatCalc/4(lb) -> qpOASES/4
  MPC_MatCalc/6(lbA) -> qpOASES/6
  Memory1/1 -> MPC_MatCalc/3(Du)
  rt1/1 -> MPC_MatCalc/2(PQ)
  GF_bio/1 -> MPC_MatCalc/6(GF)
  PQ_meas_bio/1 -> rt1/1
  MPC_MatCalc/2(F) -> qpOASES/2
  Memory2/1 -> MPC_MatCalc/4(MPCout)
  MPC_MatCalc/5(ub) -> qpOASES/5
  MPC_MatCalc/3(A) -> qpOASES/3
  rt/1 -> MPC_MatCalc/1(ref)
  MPC_MatCalc/1(Hv) -> qpOASES/1
  PQref_Bio/1 -> rt/1
  MPC_MatCalc1/7(ubA) -> qpOASES1/7
  G_Diesel/1 -> MPC_MatCalc1/5(G)
  MPC_MatCalc1/4(lb) -> qpOASES1/4
  MPC_MatCalc1/6(lbA) -> qpOASES1/6
  Memory3/1 -> MPC_MatCalc1/3(Du)
  rt3/1 -> MPC_MatCalc1/2(PQ)
  GF_Diesel/1 -> MPC_MatCalc1/6(GF)
  PQ_meas_Diesel/1 -> rt3/1
  MPC_MatCalc1/2(F) -> qpOASES1/2
  Memory4/1 -> MPC_MatCalc1/4(MPCout)
  MPC_MatCalc1/5(ub) -> qpOASES1/5
  MPC_MatCalc1/3(A) -> qpOASES1/3
  rt2/1 -> MPC_MatCalc1/1(ref)
  MPC_MatCalc1/1(Hv) -> qpOASES1/1
  PQref_Diesel/1 -> rt2/1
  [Duv_Bio] -> Memory1/1
  [Out_Bio] -> Memory2/1
  [Duv_Diesel] -> Memory3/1
  [Out_Diesel] -> Memory4/1
  qpOASES1/1 -> MPC_OutLogic1/1(duv)
  qpOASES/1 -> MPC_OutLogic/1(duv)
  MPC_OutLogic1/2(Duv) -> [Duv_Diesel]  "Delta_U"
  MPC_OutLogic/1(MPCout) -> [Out_Bio]  "mpc__out_biogen"
  MPC_OutLogic1/1(MPCout) -> [Out_Diesel]  "mpc__out"
  Mux/1 -> TrueTime Kernel/1
  MPC_OutLogic/2(Duv) -> [Duv_Bio]  "Delta_U_bio_gen"
  TrueTime Kernel/1 -> Demux/1
  Demux/2 -> MPC_DIESEL_OUT/1
  Demux/1 -> MPC_BIO_OUT/1
  [Out_Diesel] -> Mux/2
  [Out_Bio] -> Mux/1

== system uGrid_1PH_hd_ATD2/MeasureNode_I1 ==
  in : Inport
  Constant : Constant
  Product3 : Product
  Pulse Generator : DiscretePulseGenerator  PulseType=Time based  Period=50e-3  PulseWidth=50
  Pulse Generator1 : DiscretePulseGenerator  PulseType=Time based  Period=1e-4  PulseWidth=50  PhaseDelay=2e-3
  Scope : Scope
  Step : Step  Time=.5  SampleTime=0
  Switch : Switch  Criteria=u2 > Threshold  Threshold=.5
  TrueTime Receive : truetime/TrueTime Receive  nwnbr=1  receiver=4  outdim=1  triggeroutput=on  senderoutput=off  lengthoutput=off  priorityoutput=off  timestampoutput=off  signalpoweroutput=off  msgIDoutput=off
  TrueTime Send : truetime/TrueTime Send  trigger=falling  nwnbr=1  sender=3  indim=1  recsource=internal  receiver=4  lengthsource=internal  length=10000  priosource=internal  prio=1  msgIDsource=internal  msgID=0  dynamicSegment=dynamic
  Out : Outport
  wires:
  in/1 -> Product3/2
  Step/1 -> Switch/2
  Switch/1 -> Scope/1, Product3/1
  Constant/1 -> Switch/3
  Pulse Generator/1 -> Switch/1
  Pulse Generator1/1 -> TrueTime Send/2
  Product3/1 -> TrueTime Send/1
  TrueTime Receive/1 -> Out/1

== system uGrid_1PH_hd_ATD2/MeasureNode_I2 ==
  in : Inport
  Constant : Constant  Commented=on
  Product3 : Product
  Pulse Generator : DiscretePulseGenerator  Commented=on  PulseType=Time based  Period=50e-3  PulseWidth=50
  Pulse Generator1 : DiscretePulseGenerator  PulseType=Time based  Period=1e-4  PulseWidth=50  PhaseDelay=1e-3
  Step : Step  Commented=on  Time=0.4  SampleTime=0
  Step1 : Step  Time=0.4  Before=1  After=0  SampleTime=0
  Switch : Switch  Commented=on  Criteria=u2 > Threshold  Threshold=.5
  TrueTime Receive : truetime/TrueTime Receive  nwnbr=1  receiver=2  outdim=1  triggeroutput=on  senderoutput=off  lengthoutput=off  priorityoutput=off  timestampoutput=off  signalpoweroutput=off  msgIDoutput=off
  TrueTime Send : truetime/TrueTime Send  trigger=falling  nwnbr=1  sender=1  indim=1  recsource=internal  receiver=2  lengthsource=internal  length=10000  priosource=internal  prio=1  msgIDsource=internal  msgID=0  dynamicSegment=dynamic
  Out : Outport
  wires:
  in/1 -> Product3/2
  Step/1 -> Switch/2
  Constant/1 -> Switch/3
  Pulse Generator/1 -> Switch/1
  Product3/1 -> TrueTime Send/1
  TrueTime Receive/1 -> Out/1
  Pulse Generator1/1 -> TrueTime Send/2
  Step1/1 -> Product3/1

== system uGrid_1PH_hd_ATD2/MeasureNode_I3 ==
  in : Inport
  Constant : Constant
  Product3 : Product
  Pulse Generator : DiscretePulseGenerator  PulseType=Time based  Period=50e-3  PulseWidth=50
  Pulse Generator1 : DiscretePulseGenerator  PulseType=Time based  Period=1e-4  PulseWidth=50  PhaseDelay=3e-3
  Step : Step  Time=7  SampleTime=0
  Switch : Switch  Criteria=u2 > Threshold  Threshold=.5
  TrueTime Receive : truetime/TrueTime Receive  nwnbr=1  receiver=6  outdim=1  triggeroutput=on  senderoutput=off  lengthoutput=off  priorityoutput=off  timestampoutput=off  signalpoweroutput=off  msgIDoutput=off
  TrueTime Send : truetime/TrueTime Send  trigger=falling  nwnbr=1  sender=5  indim=1  recsource=internal  receiver=6  lengthsource=internal  length=10000  priosource=internal  prio=1  msgIDsource=internal  msgID=0  dynamicSegment=dynamic
  Out : Outport
  wires:
  Pulse Generator/1 -> Switch/1
  Constant/1 -> Switch/3
  Switch/1 -> Product3/1
  Step/1 -> Switch/2
  in/1 -> Product3/2
  Pulse Generator1/1 -> TrueTime Send/2
  Product3/1 -> TrueTime Send/1
  TrueTime Receive/1 -> Out/1

== system uGrid_1PH_hd_ATD2/MeasureNode_I4 ==
  in : Inport
  Constant : Constant  Commented=on
  Fcn : Fcn  Expr=u
  Multiply : Product
  Pulse Generator : DiscretePulseGenerator  Commented=on  PulseType=Time based  Period=50e-3  PulseWidth=50
  Pulse Generator1 : DiscretePulseGenerator  PulseType=Time based  Period=1e-4  PulseWidth=50  PhaseDelay=4e-3
  Step : Step  Commented=on  Time=0  SampleTime=0.25
  Step1 : Step  Time=0  SampleTime=0
  Switch : Switch  Commented=on  Criteria=u2 > Threshold  Threshold=.5
  TrueTime Receive : truetime/TrueTime Receive  nwnbr=1  receiver=8  outdim=1  triggeroutput=on  senderoutput=off  lengthoutput=off  priorityoutput=off  timestampoutput=off  signalpoweroutput=off  msgIDoutput=off
  TrueTime Send : truetime/TrueTime Send  trigger=falling  nwnbr=1  sender=7  indim=1  recsource=internal  receiver=8  lengthsource=internal  length=10000  priosource=internal  prio=1  msgIDsource=internal  msgID=0  dynamicSegment=dynamic
  Out : Outport
  wires:
  Pulse Generator/1 -> Switch/1
  Constant/1 -> Switch/3
  Step/1 -> Switch/2
  Pulse Generator1/1 -> TrueTime Send/2
  Fcn/1 -> Multiply/2
  TrueTime Receive/1 -> Out/1
  in/1 -> Fcn/1
  Multiply/1 -> TrueTime Send/1
  Step1/1 -> Multiply/1

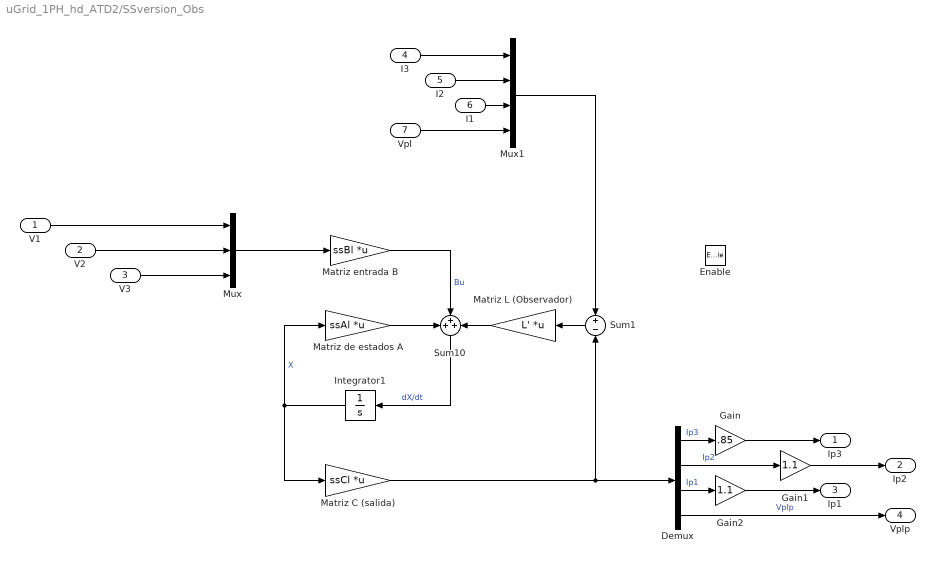
== system uGrid_1PH_hd_ATD2/SSversion_Obs ==
  V1 : Inport
  V2 : Inport  Port=2
  V3 : Inport  Port=3
  I3 : Inport  Port=4
  I2 : Inport  Port=5
  I1 : Inport  Port=6
  Vpl : Inport  Port=7
  Enable : EnablePort
  Demux : Demux
  Gain : Gain  Gain=.85
  Gain1 : Gain  Gain=1.1
  Gain2 : Gain  Gain=1.1
  Integrator1 : Integrator
  Matriz C (salida) : Gain  Gain=ssCl  Multiplication=Matrix(K*u)
  Matriz L (Observador) : Gain  Gain=L'  Multiplication=Matrix(K*u)
  Matriz de estados A : Gain  Gain=ssAl  Multiplication=Matrix(K*u)
  Matriz entrada B : Gain  Gain=ssBl  Multiplication=Matrix(K*u)
  Mux : Mux  Inputs=3
  Mux1 : Mux
  Sum1 : Sum  Inputs=+|-
  Sum10 : Sum  Inputs=+++
  Ip3 : Outport
  Ip2 : Outport  Port=2
  Ip1 : Outport  Port=3
  Vplp : Outport  Port=4
  wires:
  Matriz C (salida)/1 -> Demux/1, Sum1/2
  V1/1 -> Mux/1
  V2/1 -> Mux/2
  Demux/3 -> Gain2/1  "Ip1"
  V3/1 -> Mux/3
  Mux/1 -> Matriz entrada B/1
  Sum10/1 -> Integrator1/1  "dX/dt"
  Demux/2 -> Gain1/1  "Ip2"
  Demux/4 -> Vplp/1  "Vplp"
  Integrator1/1 -> Matriz de estados A/1, Matriz C (salida)/1  "X"
  Demux/1 -> Gain/1  "Ip3"
  Matriz de estados A/1 -> Sum10/1
  Matriz entrada B/1 -> Sum10/2  "Bu"
  I2/1 -> Mux1/2
  I3/1 -> Mux1/1
  I1/1 -> Mux1/3
  Vpl/1 -> Mux1/4
  Matriz L (Observador)/1 -> Sum10/3
  Sum1/1 -> Matriz L (Observador)/1
  Mux1/1 -> Sum1/1
  Gain/1 -> Ip3/1
  Gain1/1 -> Ip2/1
  Gain2/1 -> Ip1/1

== system uGrid_1PH_hd_ATD2/Subsystem ==
  Battery : electricdrivelib/Extra Sources/Battery  BatType=Lithium-Ion  ShowTempParam=off  ThermalPreset=no  ShowAgeParam=off  NomV=1000  NomQ=20  SOC=100  Batt_Tr=10e-3  PresetModel=off  MaxQ=1  MinV=825  FullV=1280.3859  Dis_rate=200  R=50e-3  Normal_OP=0.90435  expZone="[1188.4244    0.049130435]"  current=[6.5 13 32.5 50]  Units=Time  Tci=20  NomT=20  T2=-30  MaxQ2=4.8  FullV2=7.1  Normal_OP2=5.655  expZone2="[6.58           1]"  Rca=0.6  ti=2000  Dp=0  Neq0=0  Tsim=1e6  Ta1=25  Qeol=5.4*0.9  Reol=0.013333*1.2  Char_age=[2.3478, 3]  Dis_age=[2.3478, 10]  N1=1500  N2=10500  N3=1000  N4=1400  Ta2=45  N5=950
  Constant2 : Constant  Value=1000
  Constant4 : Constant  Value=25
  Controlled Current Source : powerlib/Electrical Sources/Controlled Current Source  Initialize=on  Source_Type=AC  Amplitude=0  Phase=0  Frequency=0  Measurements=None
  Gain3 : Gain  Gain=1/10
  PV panel1 : Subsystem
      mask Display: image('panel.jpg')
  Rcable : powerlib/Elements/Series RLC Branch  LConnTagsString=__new0  RConnTagsString=__new0  BranchType=R  Resistance=1e-3  Inductance=1e-3  SetiL0=off  InitialCurrent=0  Capacitance=1e-6  Setx0=off  InitialVoltage=0  Measurements=None
  Rin2 : powerlib/Elements/Series RLC Branch  LConnTagsString=__new0  RConnTagsString=__new0  BranchType=C  Resistance=.001  Inductance=0  SetiL0=off  InitialCurrent=0  Capacitance=1000e-6  Setx0=off  InitialVoltage=0  Measurements=None
  + : PMIOPort  Side=Left
  - : PMIOPort  Port=2  Side=Left
  Out1 : Outport
  wires:
  PV panel1/1(I) -> Gain3/1
  Gain3/1 -> Controlled Current Source/1
  Battery/1 -> Out1/1
  Constant4/1 -> PV panel1/3(Top)
  Constant2/1 -> PV panel1/2(G)
  [V] -> PV panel1/1(V)
  connections:
  Rcable/RConn1 -- +/RConn1
  Battery/LConn1 -- Controlled Current Source/RConn1 -- Rcable/LConn1 -- Rin2/LConn1
  Battery/LConn2 -- -/RConn1 -- Rin2/RConn1 -- Controlled Current Source/LConn1
